simulink model "common_2"  (R2015b)
settings: Solver=ode4  StartTime=0.0  StopTime=10  FixedStep=0.005  RelTol=1e-3
undefined symbols (not defined in the file): dq_init, g, para, q_init
settings Model: Creator=Administrator  LastModifiedBy=Administrator

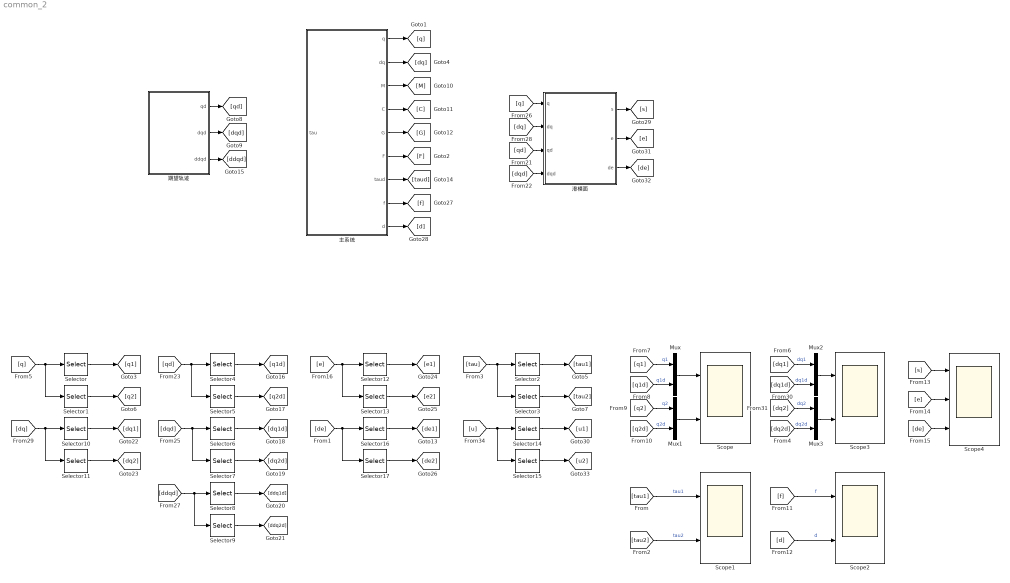
== system common_2 ==
  Mux{,1..3} (4 alike) : Mux  Inputs=2
  Scope{,1..3} (4 alike) : Scope  NumInputPorts=2
  Scope4 : Scope  NumInputPorts=3
  Selector{,2,4,6,8,10,12,14,16} (9 alike) : Selector  InputPortWidth=2  IndexOptions=Index vector (dialog)  Indices=[1]  OutputSizes=1
  Selector{1,3,5,7,9,11,13,15,17} (9 alike) : Selector  InputPortWidth=2  IndexOptions=Index vector (dialog)  Indices=[2]  OutputSizes=1
  主系统 : Subsystem
  期望轨迹 : Subsystem
  滑模面 : Subsystem
  wires:
  Selector/1 -> [q1]
  Selector1/1 -> [q2]
  [q1] -> Mux/1  "q1"
  [q1d] -> Mux/2  "q1d"
  Mux/1 -> Scope/1
  [q2] -> Mux1/1  "q2"
  [q2d] -> Mux1/2  "q2d"
  Mux1/1 -> Scope/2
  期望轨迹/1(qd) -> [qd]
  期望轨迹/2(dqd) -> [dqd]
  期望轨迹/3(ddqd) -> [ddqd]
  Selector4/1 -> [q1d]
  Selector5/1 -> [q2d]
  Selector6/1 -> [dq1d]
  Selector7/1 -> [dq2d]
  Selector8/1 -> [ddq1d]
  Selector9/1 -> [ddq2d]
  [qd] -> Selector5/1, Selector4/1
  [dqd] -> Selector7/1, Selector6/1
  [ddqd] -> Selector9/1, Selector8/1
  Selector10/1 -> [dq1]
  Selector11/1 -> [dq2]
  [q] -> Selector1/1, Selector/1
  [dq] -> Selector11/1, Selector10/1
  [dq1] -> Mux2/1  "dq1"
  [dq1d] -> Mux2/2  "dq1d"
  Mux2/1 -> Scope3/1
  [dq2] -> Mux3/1  "dq2"
  [dq2d] -> Mux3/2  "dq2d"
  Mux3/1 -> Scope3/2
  Selector13/1 -> [e2]
  [e] -> Selector13/1, Selector12/1
  Selector12/1 -> [e1]
  主系统/1(q) -> [q]
  主系统/2(dq) -> [dq]
  主系统/3(M) -> [M]
  主系统/4(C) -> [C]
  主系统/5(G) -> [G]
  [qd] -> 滑模面/3(qd)
  [dqd] -> 滑模面/4(dqd)
  [q] -> 滑模面/1(q)
  [dq] -> 滑模面/2(dq)
  滑模面/2(e) -> [e]
  滑模面/3(de) -> [de]
  主系统/6(F) -> [F]
  主系统/7(taud) -> [taud]
  Selector17/1 -> [de2]
  [de] -> Selector16/1, Selector17/1
  Selector16/1 -> [de1]
  Selector2/1 -> [tau1]
  Selector3/1 -> [tau2]
  [tau] -> Selector3/1, Selector2/1
  Selector14/1 -> [u1]
  Selector15/1 -> [u2]
  [u] -> Selector14/1, Selector15/1
  [tau1] -> Scope1/1  "tau1"
  [tau2] -> Scope1/2  "tau2"
  主系统/8(f) -> [f]
  主系统/9(d) -> [d]
  [f] -> Scope2/1  "f"
  [d] -> Scope2/2  "d"
  滑模面/1(s) -> [s]
  [s] -> Scope4/1
  [e] -> Scope4/2
  [de] -> Scope4/3

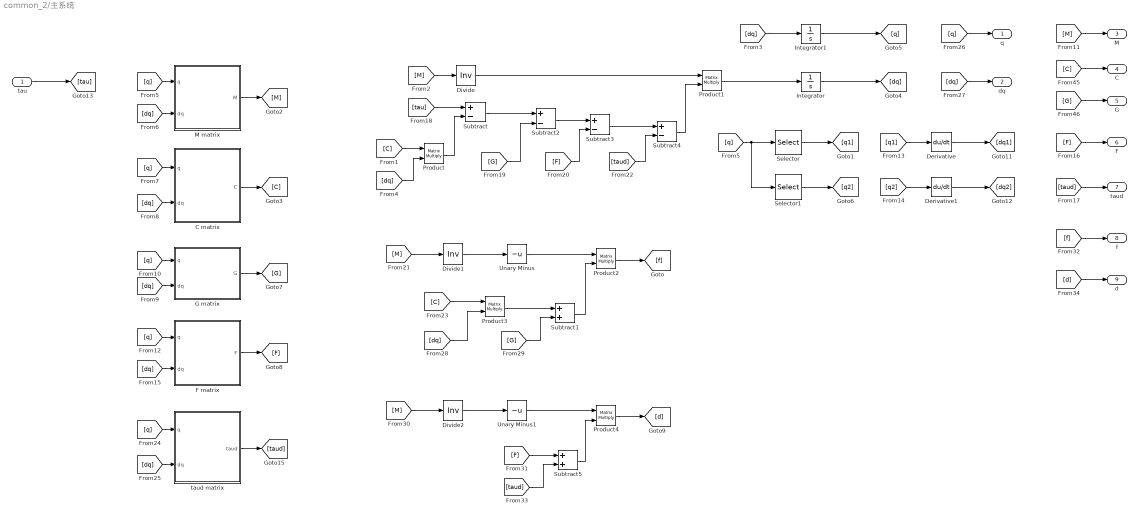
== system common_2/主系统 ==
  tau : Inport
  C matrix : Subsystem
  Derivative : Derivative
  Derivative1 : Derivative
  Divide : Product  Inputs=/  Multiplication=Matrix(*)
  Divide1 : Product  Inputs=/  Multiplication=Matrix(*)
  Divide2 : Product  Inputs=/  Multiplication=Matrix(*)
  F matrix : Subsystem
  G matrix : Subsystem
  Integrator : Integrator  InitialCondition=dq_init
  Integrator1 : Integrator  InitialCondition=q_init
  M matrix : Subsystem
  Product{,1..4} (5 alike) : Product  Multiplication=Matrix(*)
  Selector : Selector  InputPortWidth=2  IndexOptions=Index vector (dialog)  Indices=[1]  OutputSizes=1
  Selector1 : Selector  InputPortWidth=2  IndexOptions=Index vector (dialog)  Indices=[2]  OutputSizes=1
  Subtract{,2..4} (4 alike) : Sum  Inputs=+-
  Subtract1 : Sum
  Subtract5 : Sum
  Unary Minus : UnaryMinus
  Unary Minus1 : UnaryMinus
  taud matrix : Subsystem
  q : Outport
  dq : Outport  Port=2
  M : Outport  Port=3
  C : Outport  Port=4
  G : Outport  Port=5
  F : Outport  Port=6
  taud : Outport  Port=7
  f : Outport  Port=8
  d : Outport  Port=9
  wires:
  Integrator/1 -> [dq]
  [dq] -> Integrator1/1
  Integrator1/1 -> [q]
  Selector/1 -> [q1]
  Selector1/1 -> [q2]
  [q] -> Selector1/1, Selector/1
  [q1] -> Derivative/1
  Derivative/1 -> [dq1]
  [q2] -> Derivative1/1
  Derivative1/1 -> [dq2]
  [q] -> q/1
  [dq] -> dq/1
  [M] -> M/1
  [C] -> C/1
  [G] -> G/1
  [q] -> C matrix/1(q)
  [dq] -> C matrix/2(dq)
  [q] -> M matrix/1(q)
  M matrix/1(M) -> [M]
  C matrix/1(C) -> [C]
  G matrix/1(G) -> [G]
  F matrix/1(F) -> [F]
  [M] -> Divide/1
  Product1/1 -> Integrator/1
  tau/1 -> [tau]
  [q] -> G matrix/1(q)
  [q] -> F matrix/1(q)
  [dq] -> F matrix/2(dq)
  [q] -> taud matrix/1(q)
  [dq] -> taud matrix/2(dq)
  taud matrix/1(taud) -> [taud]
  [F] -> F/1
  [taud] -> taud/1
  Divide/1 -> Product1/1
  [tau] -> Subtract/1
  [C] -> Product/1
  [dq] -> Product/2
  Product/1 -> Subtract/2
  Subtract/1 -> Subtract2/1
  [G] -> Subtract2/2
  Subtract2/1 -> Subtract3/1
  [F] -> Subtract3/2
  Subtract3/1 -> Subtract4/1
  [taud] -> Subtract4/2
  Subtract4/1 -> Product1/2
  [dq] -> M matrix/2(dq)
  [dq] -> G matrix/2(dq)
  [M] -> Divide1/1
  Divide1/1 -> Unary Minus/1
  Unary Minus/1 -> Product2/1
  [C] -> Product3/1
  [dq] -> Product3/2
  Product3/1 -> Subtract1/1
  [G] -> Subtract1/2
  Subtract1/1 -> Product2/2
  Product2/1 -> [f]
  [M] -> Divide2/1
  Divide2/1 -> Unary Minus1/1
  Unary Minus1/1 -> Product4/1
  [F] -> Subtract5/1
  [taud] -> Subtract5/2
  Subtract5/1 -> Product4/2
  Product4/1 -> [d]
  [f] -> f/1
  [d] -> d/1

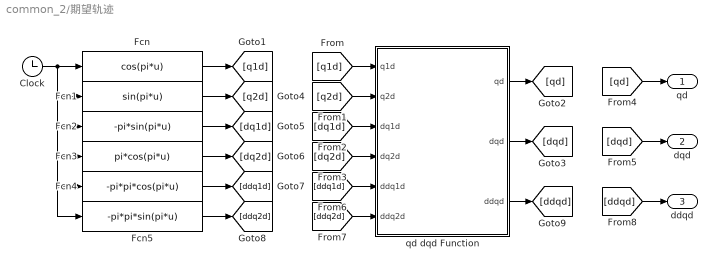
== system common_2/期望轨迹 ==
  Clock : Clock
  Fcn : Fcn  Expr=cos(pi*u)
  Fcn1 : Fcn  Expr=sin(pi*u)
  Fcn2 : Fcn  Expr=-pi*sin(pi*u)
  Fcn3 : Fcn  Expr=pi*cos(pi*u)
  Fcn4 : Fcn  Expr=-pi*pi*cos(pi*u)
  Fcn5 : Fcn  Expr=-pi*pi*sin(pi*u)
  qd dqd Function : MATLAB Function  TreatAsAtomicUnit=on
  qd : Outport
  dqd : Outport  Port=2
  ddqd : Outport  Port=3
  wires:
  qd dqd Function/2(dqd) -> [dqd]
  qd dqd Function/1(qd) -> [qd]
  Clock/1 -> Fcn5/1, Fcn4/1, Fcn3/1, Fcn2/1, Fcn1/1, Fcn/1
  Fcn/1 -> [q1d]
  Fcn1/1 -> [q2d]
  Fcn2/1 -> [dq1d]
  Fcn3/1 -> [dq2d]
  [q1d] -> qd dqd Function/1(q1d)
  [q2d] -> qd dqd Function/2(q2d)
  [dq1d] -> qd dqd Function/3(dq1d)
  [dq2d] -> qd dqd Function/4(dq2d)
  [qd] -> qd/1
  [dqd] -> dqd/1
  Fcn4/1 -> [ddq1d]
  [ddq1d] -> qd dqd Function/5(ddq1d)
  [ddq2d] -> qd dqd Function/6(ddq2d)
  qd dqd Function/3(ddqd) -> [ddqd]
  [ddqd] -> ddqd/1
  Fcn5/1 -> [ddq2d]

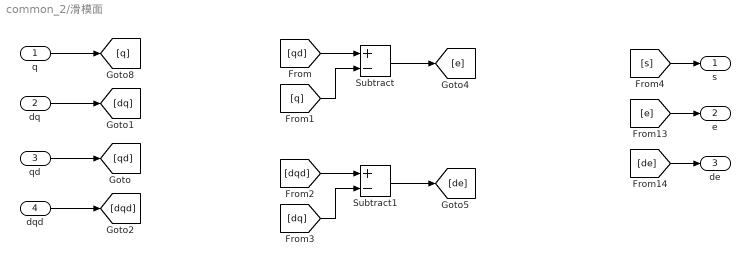
== system common_2/滑模面 ==
  q : Inport
  dq : Inport  Port=2
  qd : Inport  Port=3
  dqd : Inport  Port=4
  Subtract : Sum  Inputs=+-
  Subtract1 : Sum  Inputs=+-
  s : Outport
  e : Outport  Port=2
  de : Outport  Port=3
  wires:
  qd/1 -> [qd]
  dqd/1 -> [dqd]
  [qd] -> Subtract/1
  [q] -> Subtract/2
  Subtract/1 -> [e]
  [dqd] -> Subtract1/1
  [dq] -> Subtract1/2
  Subtract1/1 -> [de]
  q/1 -> [q]
  dq/1 -> [dq]
  [e] -> e/1
  [de] -> de/1
  [s] -> s/1

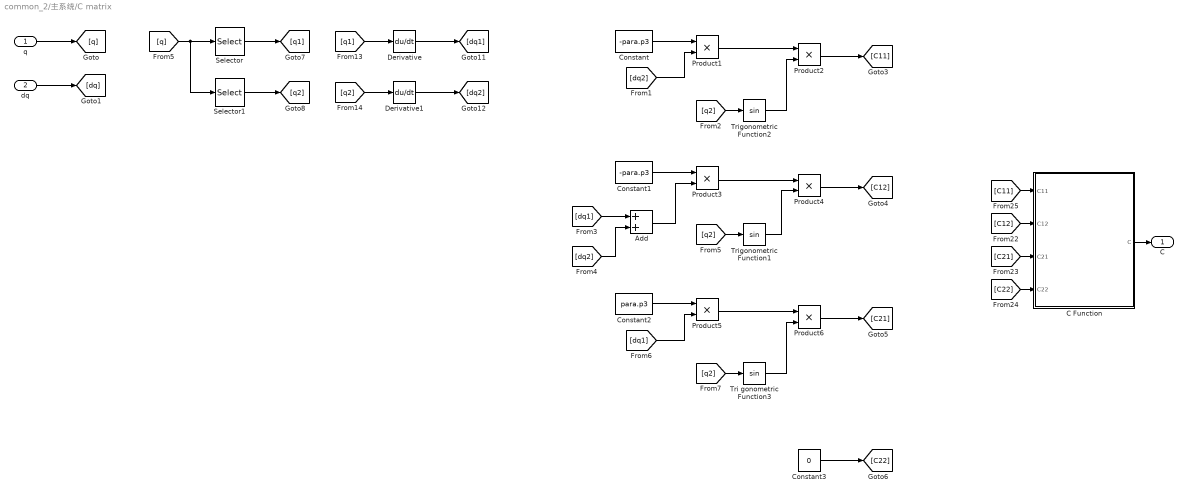
== system common_2/主系统/C matrix ==
  q : Inport
  dq : Inport  Port=2
  Add : Sum
  C Function : MATLAB Function  TreatAsAtomicUnit=on
  Constant : Constant  Value=-para.p3
  Constant1 : Constant  Value=-para.p3
  Constant2 : Constant  Value=para.p3
  Constant3 : Constant  Value=0
  Derivative : Derivative
  Derivative1 : Derivative
  Product{1..6} (6 alike) : Product
  Selector : Selector  InputPortWidth=2  IndexOptions=Index vector (dialog)  Indices=[1]  OutputSizes=1
  Selector1 : Selector  InputPortWidth=2  IndexOptions=Index vector (dialog)  Indices=[2]  OutputSizes=1
  Tri gonometric Function3 : Trigonometry
  Trigonometric Function1 : Trigonometry
  Trigonometric Function2 : Trigonometry
  C : Outport
  wires:
  [C11] -> C Function/1(C11)
  [C12] -> C Function/2(C12)
  [C21] -> C Function/3(C21)
  [C22] -> C Function/4(C22)
  C Function/1(C) -> C/1
  q/1 -> [q]
  dq/1 -> [dq]
  Constant/1 -> Product1/1
  [dq2] -> Product1/2
  Product1/1 -> Product2/1
  [q2] -> Trigonometric Function2/1
  Trigonometric Function2/1 -> Product2/2
  Selector/1 -> [q1]
  Selector1/1 -> [q2]
  [q] -> Selector1/1, Selector/1
  [q1] -> Derivative/1
  Derivative/1 -> [dq1]
  [q2] -> Derivative1/1
  Derivative1/1 -> [dq2]
  Product2/1 -> [C11]
  Constant1/1 -> Product3/1
  [dq1] -> Add/1
  [dq2] -> Add/2
  Add/1 -> Product3/2
  Product3/1 -> Product4/1
  [q2] -> Trigonometric Function1/1
  Trigonometric Function1/1 -> Product4/2
  Product4/1 -> [C12]
  Constant2/1 -> Product5/1
  [dq1] -> Product5/2
  Product5/1 -> Product6/1
  [q2] -> Tri gonometric Function3/1
  Tri gonometric Function3/1 -> Product6/2
  Product6/1 -> [C21]
  Constant3/1 -> [C22]

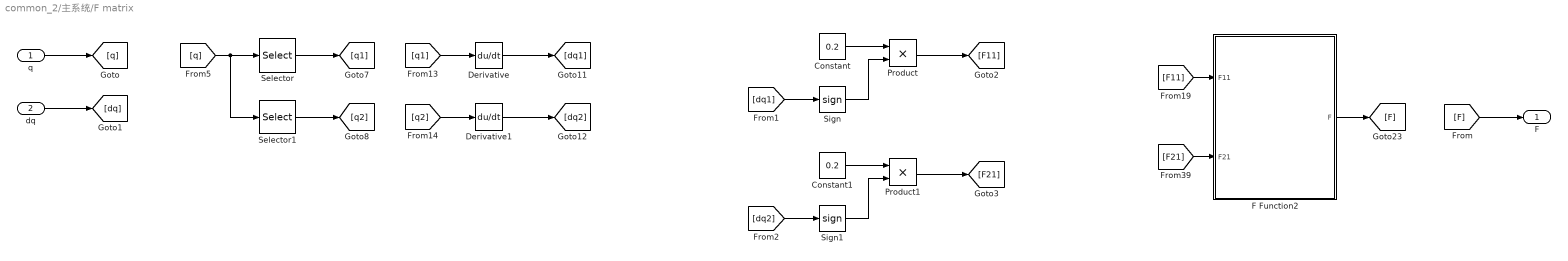
== system common_2/主系统/F matrix ==
  q : Inport
  dq : Inport  Port=2
  Constant : Constant  Value=0.2
  Constant1 : Constant  Value=0.2
  Derivative : Derivative
  Derivative1 : Derivative
  F Function2 : MATLAB Function  TreatAsAtomicUnit=on
  Product : Product
  Product1 : Product
  Selector : Selector  InputPortWidth=2  IndexOptions=Index vector (dialog)  Indices=[1]  OutputSizes=1
  Selector1 : Selector  InputPortWidth=2  IndexOptions=Index vector (dialog)  Indices=[2]  OutputSizes=1
  Sign : Signum
  Sign1 : Signum
  F : Outport
  wires:
  [F] -> F/1
  F Function2/1(F) -> [F]
  [F11] -> F Function2/1(F11)
  [F21] -> F Function2/2(F21)
  q/1 -> [q]
  dq/1 -> [dq]
  Selector/1 -> [q1]
  Selector1/1 -> [q2]
  [q] -> Selector1/1, Selector/1
  [q1] -> Derivative/1
  Derivative/1 -> [dq1]
  [q2] -> Derivative1/1
  Derivative1/1 -> [dq2]
  Constant/1 -> Product/1
  Sign/1 -> Product/2
  [dq1] -> Sign/1
  Product/1 -> [F11]
  Constant1/1 -> Product1/1
  Sign1/1 -> Product1/2
  [dq2] -> Sign1/1
  Product1/1 -> [F21]

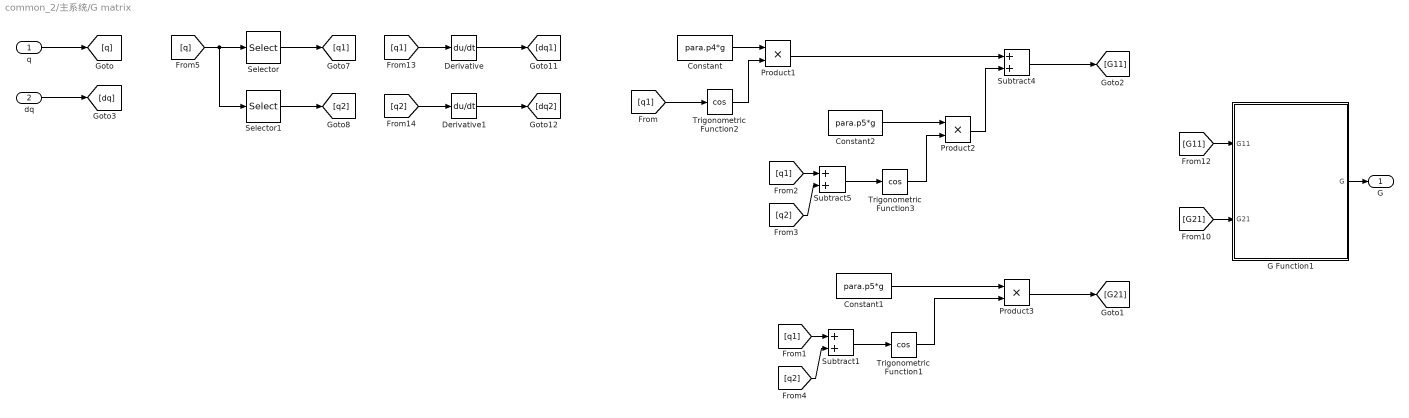
== system common_2/主系统/G matrix ==
  q : Inport
  dq : Inport  Port=2
  Constant : Constant  Value=para.p4*g
  Constant1 : Constant  Value=para.p5*g
  Constant2 : Constant  Value=para.p5*g
  Derivative : Derivative
  Derivative1 : Derivative
  G Function1 : MATLAB Function  TreatAsAtomicUnit=on
  Product1 : Product
  Product2 : Product
  Product3 : Product
  Selector : Selector  InputPortWidth=2  IndexOptions=Index vector (dialog)  Indices=[1]  OutputSizes=1
  Selector1 : Selector  InputPortWidth=2  IndexOptions=Index vector (dialog)  Indices=[2]  OutputSizes=1
  Subtract1 : Sum
  Subtract4 : Sum
  Subtract5 : Sum
  Trigonometric Function1 : Trigonometry  Operator=cos
  Trigonometric Function2 : Trigonometry  Operator=cos
  Trigonometric Function3 : Trigonometry  Operator=cos
  G : Outport
  wires:
  [G11] -> G Function1/1(G11)
  [G21] -> G Function1/2(G21)
  G Function1/1(G) -> G/1
  Constant/1 -> Product1/1
  Trigonometric Function2/1 -> Product1/2
  [q1] -> Trigonometric Function2/1
  Product1/1 -> Subtract4/1
  Constant2/1 -> Product2/1
  Subtract5/1 -> Trigonometric Function3/1
  [q1] -> Subtract5/1
  [q2] -> Subtract5/2
  Trigonometric Function3/1 -> Product2/2
  Product2/1 -> Subtract4/2
  Subtract4/1 -> [G11]
  Constant1/1 -> Product3/1
  Subtract1/1 -> Trigonometric Function1/1
  [q1] -> Subtract1/1
  [q2] -> Subtract1/2
  Trigonometric Function1/1 -> Product3/2
  Product3/1 -> [G21]
  q/1 -> [q]
  dq/1 -> [dq]
  Selector/1 -> [q1]
  Selector1/1 -> [q2]
  [q] -> Selector1/1, Selector/1
  [q1] -> Derivative/1
  Derivative/1 -> [dq1]
  [q2] -> Derivative1/1
  Derivative1/1 -> [dq2]

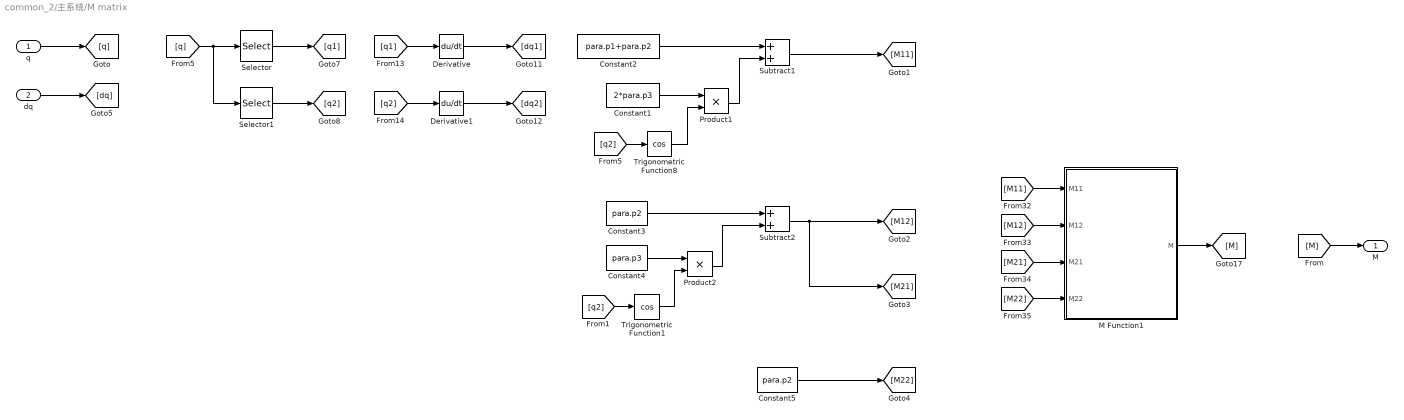
== system common_2/主系统/M matrix ==
  q : Inport
  dq : Inport  Port=2
  Constant1 : Constant  Value=2*para.p3
  Constant2 : Constant  Value=para.p1+para.p2
  Constant3 : Constant  Value=para.p2
  Constant4 : Constant  Value=para.p3
  Constant5 : Constant  Value=para.p2
  Derivative : Derivative
  Derivative1 : Derivative
  M Function1 : MATLAB Function  TreatAsAtomicUnit=on
  Product1 : Product
  Product2 : Product
  Selector : Selector  InputPortWidth=2  IndexOptions=Index vector (dialog)  Indices=[1]  OutputSizes=1
  Selector1 : Selector  InputPortWidth=2  IndexOptions=Index vector (dialog)  Indices=[2]  OutputSizes=1
  Subtract1 : Sum
  Subtract2 : Sum
  Trigonometric Function1 : Trigonometry  Operator=cos
  Trigonometric Function8 : Trigonometry  Operator=cos
  M : Outport
  wires:
  M Function1/1(M) -> [M]
  [M11] -> M Function1/1(M11)
  [M12] -> M Function1/2(M12)
  [M21] -> M Function1/3(M21)
  [M22] -> M Function1/4(M22)
  [q2] -> Trigonometric Function8/1
  [M] -> M/1
  Constant2/1 -> Subtract1/1
  Constant1/1 -> Product1/1
  Trigonometric Function8/1 -> Product1/2
  Product1/1 -> Subtract1/2
  Subtract2/1 -> [M21], [M12]
  Constant5/1 -> [M22]
  Subtract1/1 -> [M11]
  Constant3/1 -> Subtract2/1
  Constant4/1 -> Product2/1
  [q2] -> Trigonometric Function1/1
  Trigonometric Function1/1 -> Product2/2
  Product2/1 -> Subtract2/2
  q/1 -> [q]
  dq/1 -> [dq]
  Selector/1 -> [q1]
  Selector1/1 -> [q2]
  [q] -> Selector1/1, Selector/1
  [q1] -> Derivative/1
  Derivative/1 -> [dq1]
  [q2] -> Derivative1/1
  Derivative1/1 -> [dq2]

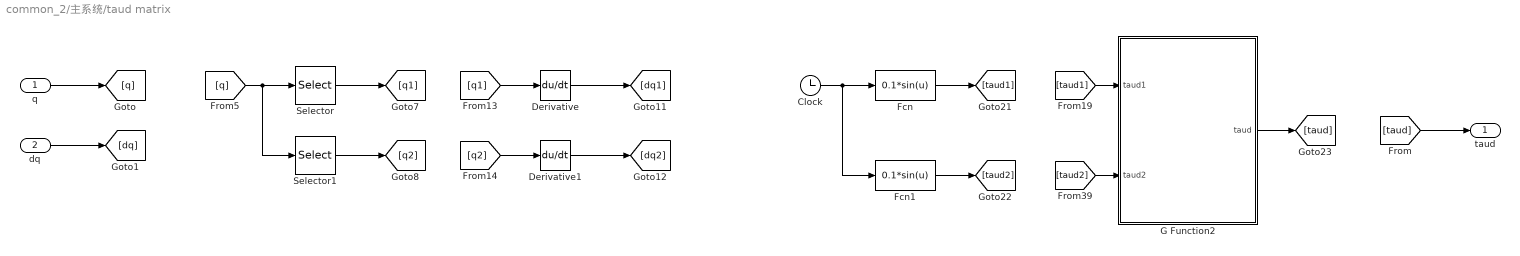
== system common_2/主系统/taud matrix ==
  q : Inport
  dq : Inport  Port=2
  Clock : Clock
  Derivative : Derivative
  Derivative1 : Derivative
  Fcn : Fcn  Expr=0.1*sin(u)
  Fcn1 : Fcn  Expr=0.1*sin(u)
  G Function2 : MATLAB Function  TreatAsAtomicUnit=on
  Selector : Selector  InputPortWidth=2  IndexOptions=Index vector (dialog)  Indices=[1]  OutputSizes=1
  Selector1 : Selector  InputPortWidth=2  IndexOptions=Index vector (dialog)  Indices=[2]  OutputSizes=1
  taud : Outport
  wires:
  [taud2] -> G Function2/2(taud2)
  [taud1] -> G Function2/1(taud1)
  G Function2/1(taud) -> [taud]
  [taud] -> taud/1
  q/1 -> [q]
  dq/1 -> [dq]
  Selector/1 -> [q1]
  Selector1/1 -> [q2]
  [q] -> Selector1/1, Selector/1
  [q1] -> Derivative/1
  Derivative/1 -> [dq1]
  [q2] -> Derivative1/1
  Derivative1/1 -> [dq2]
  Clock/1 -> Fcn1/1, Fcn/1
  Fcn/1 -> [taud1]
  Fcn1/1 -> [taud2]

== matlab function common_2/期望轨迹/qd dqd Function ==
  data: q1d input; qd output; q2d input; dq1d input; dq2d input; dqd output; ddq1d input; ddq2d input; ddqd output
function [qd,dqd,ddqd]= fcn(q1d,q2d,dq1d,dq2d,ddq1d,ddq2d)
%#codegen

qd   = [q1d;q2d];
dqd  = [dq1d;dq2d];
ddqd = [ddq1d;ddq2d];

== matlab function common_2/主系统/G matrix/G Function1 ==
  data: G11 input; G output; G21 input
function G = fcn(G11,G21)
%#codegen

G = [G11;G21];

== matlab function common_2/主系统/C matrix/C Function ==
  data: C11 input; C output; C12 input; C21 input; C22 input
function C = fcn(C11,C12,C21,C22)
%#codegen

C = [C11 C12;C21 C22];

== matlab function common_2/主系统/M matrix/M Function1 ==
  data: M11 input; M output; M12 input; M21 input; M22 input
function M = fcn(M11,M12,M21,M22)
%#codegen

M = [M11 M12;M21 M22];

== matlab function common_2/主系统/F matrix/F Function2 ==
  data: F11 input; F output; F21 input
function F = fcn(F11,F21)
%#codegen

F = [F11;F21];

== matlab function common_2/主系统/taud matrix/G Function2 ==
  data: taud1 input; taud output; taud2 input
function taud = fcn(taud1,taud2)
%#codegen

taud = [taud1;taud2];
